simulink model "washing_module"  (R2024b)
settings: Solver=VariableStepAuto  StartTime=0.0  StopTime=inf  RelTol=1e-3
settings Model: Creator=sunil  LastModifiedBy=91636

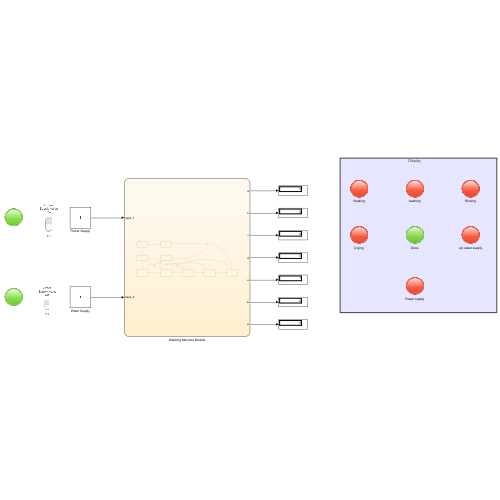
[thumbnail: Simulink's stored preview of the top-level diagram]
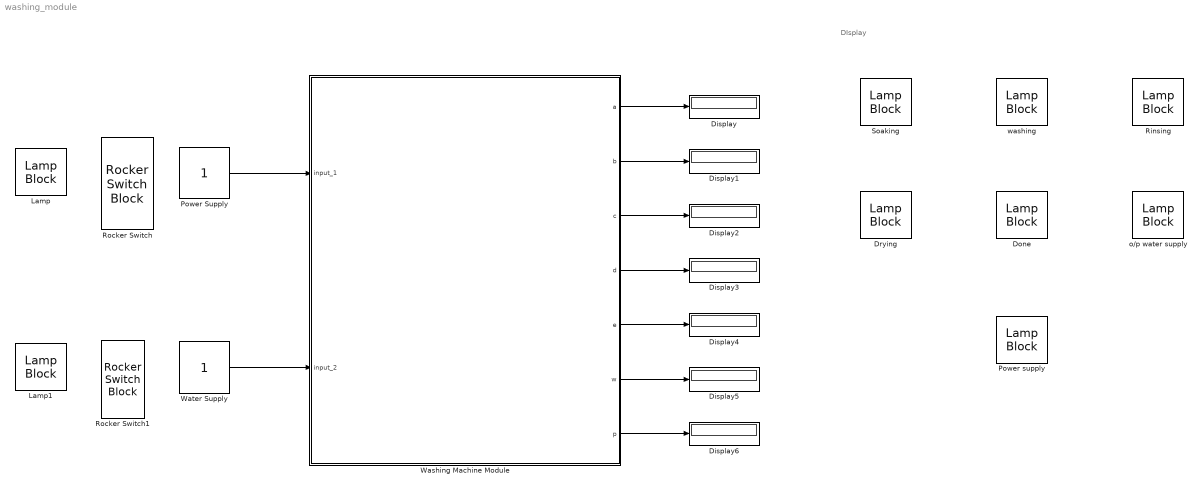
== system washing_module ==
  note: DIsplay
  Display{,1..6} (7 alike) : Display
  Done : LampBlock  LabelPosition=Hide
  Drying : LampBlock  LabelPosition=Hide
  Lamp : LampBlock  LabelPosition=Hide
  Lamp1 : LampBlock  LabelPosition=Hide
  Power Supply : Constant
  Power supply : LampBlock  LabelPosition=Hide
  Rinsing : LampBlock  LabelPosition=Hide
  Rocker Switch : RockerSwitchBlock
      settings: Values={{'Off', 'On'}, [0 1]}
  Rocker Switch1 : RockerSwitchBlock
      settings: Values={{'Off', 'On'}, [0 1]}
  Soaking : LampBlock  LabelPosition=Hide
  Washing Machine Module : Stateflow chart  TreatAsAtomicUnit=on
  Water Supply : Constant
  o/p water supply : LampBlock  LabelPosition=Hide
  washing : LampBlock  LabelPosition=Hide
  wires:
  Washing Machine Module/3(c) -> Display2/1
  Washing Machine Module/4(d) -> Display3/1
  Washing Machine Module/5(e) -> Display4/1
  Washing Machine Module/6(w) -> Display5/1
  Washing Machine Module/7(p) -> Display6/1
  Washing Machine Module/1(a) -> Display/1
  Power Supply/1 -> Washing Machine Module/1(input_1)
  Water Supply/1 -> Washing Machine Module/2(input_2)
  Washing Machine Module/2(b) -> Display1/1

== stateflow chart washing_module/Washing Machine Module ==
  state Power_suply_ON
    entry:
    if (input_1==1)
    p=1
    end
  state Power_supply_OFF
  state Water_Supply_ON
    entry:
    if (input_2==1)
    w=1
    end
  state Water_Supply_Off
  state Soaking
    entry:
    a=1
    exit:
    a=0
  state Washing
    entry:
    b=1
    exit:
    b=0
  state Rinse
    entry: c=1
    exit: c=0;
    exit: w=0;
  state Dryer
    entry: d=1;
    exit: d=0;
  state Done
    entry: e=1
    exit: p=0
  (default) -> Power_suply_ON
  (junction 21) -> Power_supply_OFF
  Done -> (junction 21) [order 1]
  Power_suply_ON -> Power_supply_OFF [order 1] : [input_1==0]
  Water_Supply_Off -> (junction 21)
  Power_suply_ON -> Water_Supply_ON [order 2] : [input_1==1]
  Water_Supply_ON -> Water_Supply_Off [order 1] : [input_2==0]
  Done -> (junction 53) [order 2] : [input_2==0||input_1==0]
  Water_Supply_ON -> Soaking [order 2] : [input_2==1]
  (junction 62) -> Water_Supply_Off : [input_2==0||input_1==0]
  (junction 50) -> (junction 62) : [input_2==0||input_1==0]
  (junction 53) -> (junction 62) : [input_2==0||input_1==0]
  Dryer -> (junction 52) [order 2] : [input_2==0||input_1==0]
  (junction 52) -> (junction 53) : [input_2==0||input_1==0]
  Soaking -> (junction 50) [order 2] : [input_2==0||input_1==0]
  Rinse -> (junction 52) [order 2] : [input_2==0||input_1==0]
  Washing -> (junction 50) [order 2] : [input_2==0||input_1==0]
  Washing -> Rinse [order 1] : [after(5,sec)]
  Rinse -> Dryer [order 1] : [after(5,sec)]
  Dryer -> Done [order 1] : [after(5,sec)]
  Soaking -> Washing [order 1] : [after(5,sec)]
  data: input_1 input; input_2 input; a output; b output; c output; d output; e output; w output; p output
